simulink library "demo_lib_sys"  (R2024a)
settings: Solver=VariableStepAuto  StartTime=0.0  StopTime=10.0  RelTol=1e-3
settings Model: Creator=luka  LastModifiedBy=luka

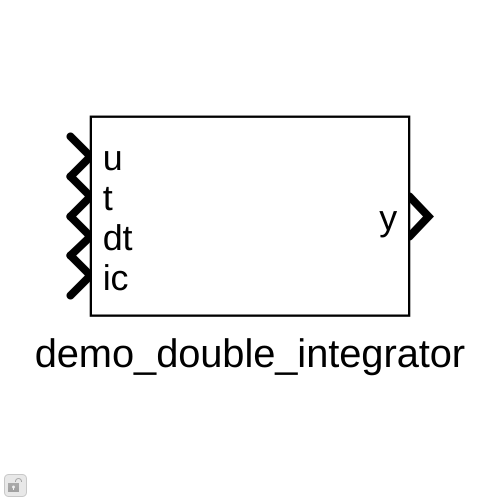
[thumbnail: Simulink's stored preview of the top-level diagram]
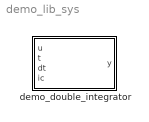
== system demo_lib_sys ==
  demo_double_integrator : Subsystem  Tag=__cs_slx_sys;  mask{k1=0, k2=0, iid__=[0], pid__=[100 101 109 111 95 100 111 117 98 108 101 95 105 110 116 101 103 114 97 116 111 114 58 100 101 109 111 95 108 105 98], params_struct_name=}
      mask DialogControl params Prompt: Parameters

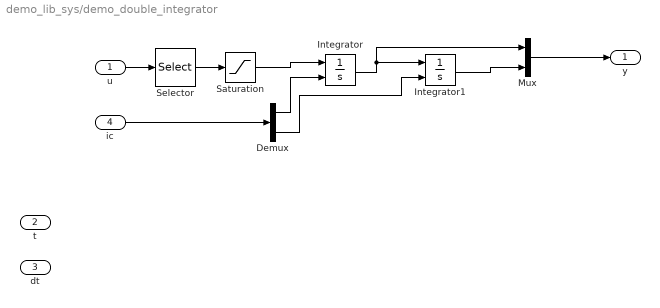
== system demo_lib_sys/demo_double_integrator ==
  u : Inport  PortDimensions=3
  t : Inport  Port=2
  dt : Inport  Port=3
  ic : Inport  Port=4
  Demux : Demux  Outputs=2
  Integrator : Integrator  InitialConditionSource=external
  Integrator1 : Integrator  InitialConditionSource=external
  Mux : Mux  Inputs=2
  Saturation : Saturate  UpperLimit=1  LowerLimit=-1
  Selector : Selector  InputPortWidth=3  IndexOptions=Index vector (dialog)  Indices=[1]  OutputSizes=1
  y : Outport  PortDimensions=2
  wires:
  Demux/2 -> Integrator1/2
  Demux/1 -> Integrator/2
  ic/1 -> Demux/1
  Mux/1 -> y/1
  Saturation/1 -> Integrator/1
  Integrator1/1 -> Mux/2
  Integrator/1 -> Integrator1/1, Mux/1
  Selector/1 -> Saturation/1
  u/1 -> Selector/1
